simulink model "ArduinoMKRTemplate"  (R2021b)
settings: Solver=FixedStepAuto  StartTime=0.0  StopTime=inf  RelTol=1e-3  EnableMultiTasking=on
libraries: arduinomotorcarrierlib x4, arduinowifilib x2, simulink x1
settings Model: ExtModeTrigDuration=2  Creator=bkhusain  LastModifiedBy=cirie
settings SolverCC: AlgebraicLoopSolver=TrustRegion
settings OptimizationCC: EnhancedBackFolding=on  PassReuseOutputArgsAs=Individual arguments  ZeroExternalMemoryAtStartup=off  ZeroInternalMemoryAtStartup=off  MaxStackSize=64  OptimizeBlockOrder=speed  DifferentSizesBufferReuse=on  OptimizationCustomize=off  EfficientTunableParamExpr=on
settings DebuggingCC: ParameterTunabilityLossMsg=error  SFMachineParentedDataDiag=warning
settings HardwareCC: ProdBitPerPointer=32  ProdBitPerSizeT=32  ProdBitPerPtrDiffT=32  ProdLargestAtomicInteger=Long  ProdLargestAtomicFloat=Double  ProdWordSize=32  ProdHWDeviceType=ARM Compatible->ARM Cortex
settings SFSimCC: MATLABDynamicMemAlloc=off
settings RTWCC: Description=Embedded Coder  SystemTargetFile=ert.tlc  HardwareBoard=Arduino MKR WiFi 1010  TemplateMakefile=ert_default_tmf  Toolchain=Arduino ARM  BuildConfiguration=Faster Runs
settings CodeAppCC: ForceParamTrailComments=on  IgnoreCustomStorageClasses=off  OperatorAnnotations=on  SimulinkDataObjDesc=on  SFDataObjDesc=on  InsertBlockDesc=on
settings ERTTargetCC: SupportContinuousTime=on  SupportVariableSizeSignals=on  ExtModeTransport=3  ExtModeStaticAlloc=on  ExtModeStaticAllocSize=8192  ExtModeMexFile=ext_xcp  ExtModeIntrfLevel=Level2 - Open

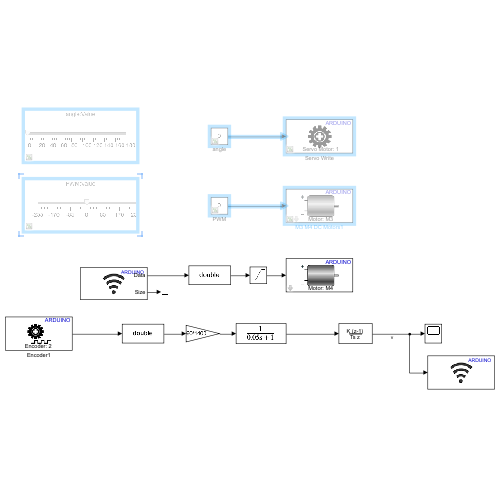
[thumbnail: Simulink's stored preview of the top-level diagram]
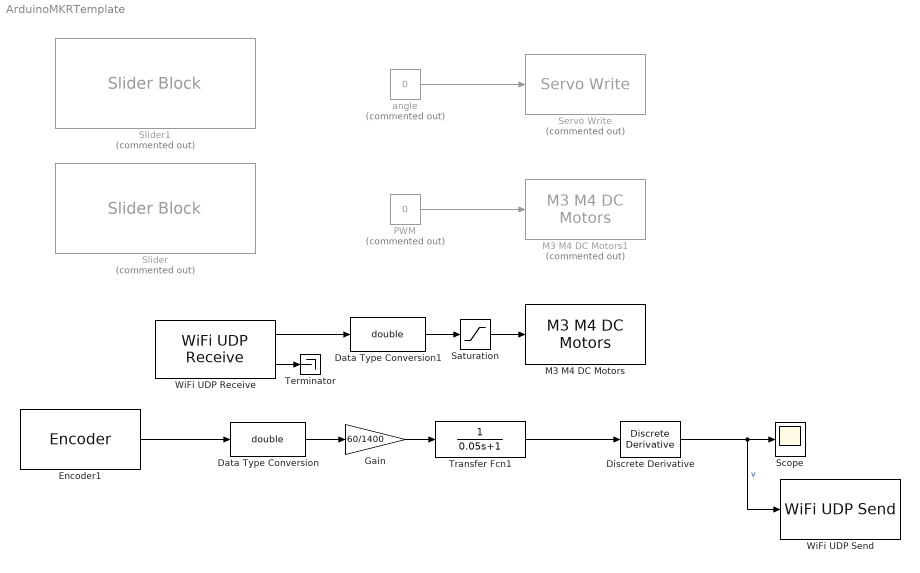
== system ArduinoMKRTemplate ==
  Data Type Conversion : DataTypeConversion  OutDataTypeStr=double
  Data Type Conversion1 : DataTypeConversion  OutDataTypeStr=double
  Discrete Derivative : simulink/Discrete/Discrete Derivative  gainval=1.0  ICPrevScaledInput=0.0  OutMin=[]  OutMax=[]  OutDataType=fixdt(1, 16)  OutScaling=2^-10  DoSatur=off
  Encoder1 : arduinomotorcarrierlib/Encoder  SlaveAddress=uint8( hex2dec( '66' ) )  blockPlatform=ARDUINO  Encoder=2  ShowSpeed=off  ResetOption=on  SampleTime=0.05
      settings: SourceProductBaseCode=ARDUINO
  Gain : Gain  Gain=60/1400
  M3 M4 DC Motors : arduinomotorcarrierlib/M3 M4 DC Motors  MotorNumber=M4  forwardPinNumber=4  reversePinNumber=5
      settings: SourceProductBaseCode=ARDUINO
  M3 M4 DC Motors1 : arduinomotorcarrierlib/M3 M4 DC Motors  Commented=on  MotorNumber=M3  forwardPinNumber=3  reversePinNumber=2
      settings: SourceProductBaseCode=ARDUINO
  PWM : Constant  Commented=on  Value=0
  Saturation : Saturate  UpperLimit=255  LowerLimit=-255
  Scope : Scope
  Servo Write : arduinomotorcarrierlib/Servo Write  Commented=on  SlaveAddress=uint8( hex2dec( '66' ) )  blockPlatform=ARDUINO  MotorNumber=1  MotorCarrierPWMFreq=100
      settings: SourceProductBaseCode=ARDUINO
  Slider : SliderBlock  Commented=on  ScaleMin=-255  ScaleMax=255
  Slider1 : SliderBlock  Commented=on  ScaleMax=180
  Terminator : Terminator
  Transfer Fcn1 : TransferFcn  Denominator=[0.05 1]
  WiFi UDP Receive : arduinowifilib/WiFi UDP Receive  localport=50001  DataType=uint8  DataLength=1  SampleTime_=0.1  wifiUDPIndex=0  blockPlatform=ARDUINO  isARMArch=false
      settings: SourceProductBaseCode=ARDUINO
  WiFi UDP Send : arduinowifilib/WiFi UDP Send  remoteIPOctetString=192.168.8.120  remoteport=50002  localport=50001  remoteipoctet1=192  remoteipoctet2=168  remoteipoctet3=1  remoteipoctet4=2  wifiUDPIndex=0  blockPlatform=ARDUINO  isARMArch=false
      settings: SourceProductBaseCode=ARDUINO
  angle : Constant  Commented=on  Value=0
  wires:
  Saturation/1 -> M3 M4 DC Motors/1
  Encoder1/1 -> Data Type Conversion/1
  Transfer Fcn1/1 -> Discrete Derivative/1
  Gain/1 -> Transfer Fcn1/1
  Data Type Conversion/1 -> Gain/1
  Discrete Derivative/1 -> WiFi UDP Send/1, Scope/1  "v"
  PWM/1 -> M3 M4 DC Motors1/1
  angle/1 -> Servo Write/1
  Data Type Conversion1/1 -> Saturation/1
  WiFi UDP Receive/1 -> Data Type Conversion1/1
  WiFi UDP Receive/2 -> Terminator/1
